simulink model "Buck_Boost_Converter"  (R2020a)
settings: Solver=VariableStepAuto  StartTime=0.0  StopTime=10.0  RelTol=1e-3
libraries: powerlib x15
settings Model: Creator=rajgo  LastModifiedBy=rajgo

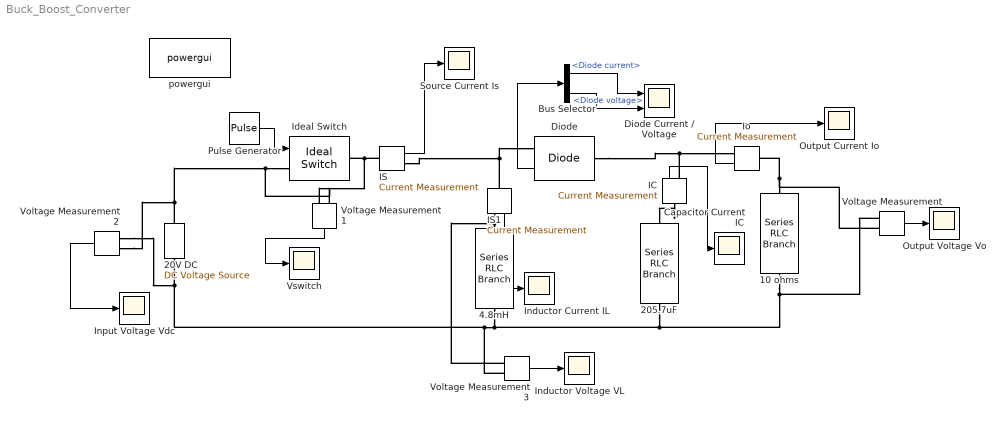
== system Buck_Boost_Converter ==
  10 ohms : powerlib/Elements/Series RLC Branch  LConnTagsString=__new0  RConnTagsString=__new0  BranchType=R  Resistance=10  Inductance=1e-3  SetiL0=off  InitialCurrent=0  Capacitance=1e-6  Setx0=off  InitialVoltage=0  Measurements=None
  205.7uF : powerlib/Elements/Series RLC Branch  LConnTagsString=__new0  RConnTagsString=__new0  BranchType=C  Resistance=1  Inductance=1e-3  SetiL0=off  InitialCurrent=0  Capacitance=205.71e-6  Setx0=off  InitialVoltage=0  Measurements=None
  20V DC : powerlib/Electrical Sources/DC Voltage Source  Amplitude=20  Measurements=None
  4.8mH : powerlib/Elements/Series RLC Branch  LConnTagsString=__new0  RConnTagsString=__new0  BranchType=L  Resistance=1  Inductance=4.8e-3  SetiL0=off  InitialCurrent=0  Capacitance=1e-6  Setx0=off  InitialVoltage=0  Measurements=None
  Bus Selector : BusSelector  OutputSignals=Diode current,Diode voltage
  Capacitor Current IC : Scope
  Diode : powerlib/Power Electronics/Diode  Ron=0.000000000001  Lon=0  Vf=0  IC=0  UseSnubber=0  Rs=inf  Cs=0  Measurements=on
  Diode Current / Voltage : Scope  NumInputPorts=2
  IC : powerlib/Measurements/Current Measurement  PhasorSimulation=off  OutputType=Complex  PSBequivalent=0
  IS : powerlib/Measurements/Current Measurement  PhasorSimulation=off  OutputType=Complex  PSBequivalent=0
  IS1 : powerlib/Measurements/Current Measurement  PhasorSimulation=off  OutputType=Complex  PSBequivalent=0
  Ideal Switch : powerlib/Power Electronics/Ideal Switch  Ron=0.000000000001  Lon=0  IC=0  Rs=0  Cs=0  Measurements=off
  Inductor Current IL : Scope
  Inductor Voltage VL : Scope
  Input Voltage Vdc : Scope
  Io : powerlib/Measurements/Current Measurement  PhasorSimulation=off  OutputType=Complex  PSBequivalent=0
  Output Current Io : Scope
  Output Voltage Vo : Scope
  Pulse Generator : DiscretePulseGenerator  PulseType=Time based  Amplitude=10  Period=1/5000  PulseWidth=30
  Source Current Is : Scope
  Voltage Measurement{,1..3} (4 alike) : powerlib/Measurements/Voltage Measurement  PhasorSimulation=off  OutputType=Complex  PSBequivalent=0
  Vswitch : Scope
  powergui : powerlib/powergui  Priority=1  SimulationMode=Continuous  SampleTime=50e-6  frequency=60  Iterations=50  frequencyindice=0  Pbase=100e6  ErrMax=1e-4  UnitsV=kV  UnitsW=MW  buscounter=0  FunctionMessages=off  echomessages=off  EnableUseOfTLC=off  CurrentSourceSwitches=off  DisableSnubberDevices=off  DisableRonSwitches=off  DisableVfSwitches=off  DisplayEquations=off  AutomaticDiscreteSolvers=off  SolverType=Tustin/Backward Euler (TBE)  Interpol=off  ExternalGateDelay=off  methode=off  Ts=100  x0status=blocks  SPID=on  SwTol=0  HookPort=off  NonlinearTolerance=1e-4  nMaxIteration=100  ContinueOnMaxIteration=off  RestoreLinks=warning  ResistiveCurrentMeasurement=off  Frange=[0:2:500]  Ylog=off  Xlog=on  ShowGrid=off  save=off  variable=ZData  structure=0  ZoomFFT=off  StartTime=0.0  cycles=1  DisplayStyle=1  fundamental=60  FreqAxis=off  MaxFrequency=1000  frequencyindicesteady=1  RmsSteady=1  display=off
  wires:
  Voltage Measurement/1 -> Output Voltage Vo/1
  Pulse Generator/1 -> Ideal Switch/1
  IS/1 -> Source Current Is/1
  Voltage Measurement1/1 -> Vswitch/1
  Voltage Measurement2/1 -> Input Voltage Vdc/1
  IS1/1 -> Inductor Current IL/1
  Voltage Measurement3/1 -> Inductor Voltage VL/1
  Diode/1 -> Bus Selector/1
  Bus Selector/1 -> Diode Current / Voltage/1  "<Diode current>"
  Bus Selector/2 -> Diode Current / Voltage/2  "<Diode voltage>"
  IC/1 -> Capacitor Current IC/1
  Io/1 -> Output Current Io/1
  connections:
  20V DC/RConn1 -- Voltage Measurement1/LConn1 -- Ideal Switch/LConn1 -- Voltage Measurement2/LConn1
  IS/RConn1 -- IS1/LConn1 -- Diode/RConn1
  Voltage Measurement/LConn2 -- Io/LConn1 -- 10 ohms/LConn1
  10 ohms/RConn1 -- Voltage Measurement/LConn1 -- Voltage Measurement3/LConn2 -- Voltage Measurement2/LConn2 -- 20V DC/LConn1 -- 4.8mH/RConn1 -- 205.7uF/RConn1
  IS/LConn1 -- Voltage Measurement1/LConn2 -- Ideal Switch/RConn1
  IS1/RConn1 -- Voltage Measurement3/LConn1 -- 4.8mH/LConn1
  Diode/LConn1 -- IC/RConn1 -- Io/RConn1
  IC/LConn1 -- 205.7uF/LConn1
